simulink model "cinematica_inversa"  (R2017b)
settings: Solver=VariableStepAuto  StartTime=0.0  StopTime=10.0  RelTol=1e-3
undefined symbols (not defined in the file): b
settings Model: Creator=jorgeluis  LastModifiedBy=jorgeluis

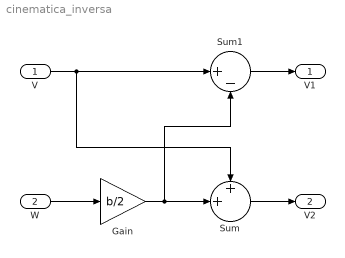
== system cinematica_inversa ==
  V : Inport
  W : Inport  Port=2
  Gain : Gain  Gain=b/2
  Sum : Sum  Inputs=++|
  Sum1 : Sum  Inputs=|+-
  V1 : Outport
  V2 : Outport  Port=2
  wires:
  W/1 -> Gain/1
  Gain/1 -> Sum1/2, Sum/2
  Sum/1 -> V2/1
  Sum1/1 -> V1/1
  V/1 -> Sum/1, Sum1/1
